simulink model "fangzhen"  (R2022a)
settings: Solver=FixedStepAuto  StartTime=0.0  StopTime=1  FixedStep=0.001  RelTol=1e-3
settings Model: Creator=Userx  LastModifiedBy=Userx

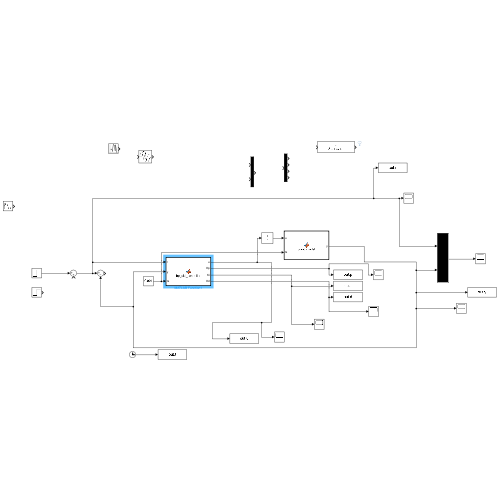
[thumbnail: Simulink's stored preview of the top-level diagram]
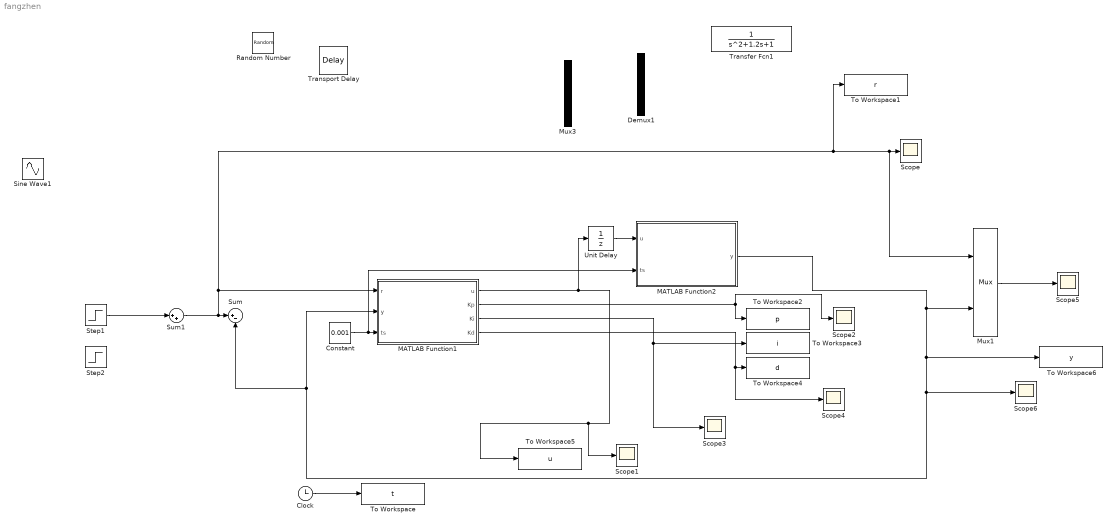
== system fangzhen ==
  Clock : Clock
  Constant : Constant  Value=0.001
  Demux1 : Demux
  MATLAB Function1 : MATLAB Function  TreatAsAtomicUnit=on
  MATLAB Function2 : MATLAB Function  TreatAsAtomicUnit=on
  Mux1 : Mux  Inputs=2
  Mux3 : Mux  Inputs=2
  Random Number : RandomNumber  Variance=0.05  SampleTime=0.1
  Scope{,1..6} (7 alike) : Scope
  Sine Wave1 : Sin  Frequency=5  SampleTime=0
  Step1 : Step  Time=0  SampleTime=0
  Step2 : Step  Time=200  SampleTime=0
  Sum : Sum  Inputs=|+-
  Sum1 : Sum  Inputs=|++
  To Workspace : ToWorkspace  VariableName=t  SampleTime=-1
  To Workspace1 : ToWorkspace  VariableName=r  SampleTime=-1
  To Workspace2 : ToWorkspace  VariableName=p  SampleTime=-1
  To Workspace3 : ToWorkspace  VariableName=i  SampleTime=-1
  To Workspace4 : ToWorkspace  VariableName=d  SampleTime=-1
  To Workspace5 : ToWorkspace  VariableName=u  SampleTime=-1
  To Workspace6 : ToWorkspace  VariableName=y  SampleTime=-1
  Transfer Fcn1 : TransferFcn  Denominator=[1 1.2 1]
  Transport Delay : TransportDelay  DelayTime=0.5
  Unit Delay : UnitDelay  SampleTime=-1  HasFrameUpgradeWarning=on
  wires:
  Mux1/1 -> Scope5/1
  MATLAB Function1/2(Kp) -> Scope2/1, To Workspace2/1
  MATLAB Function1/3(Ki) -> Scope3/1, To Workspace3/1
  MATLAB Function1/4(Kd) -> Scope4/1, To Workspace4/1
  Clock/1 -> To Workspace/1
  Sum1/1 -> MATLAB Function1/1(r), To Workspace1/1, Mux1/1, Scope/1, Sum/1
  MATLAB Function2/1(y) -> MATLAB Function1/2(y), Sum/2, Scope6/1, To Workspace6/1, Mux1/2
  Step1/1 -> Sum1/1
  MATLAB Function1/1(u) -> Unit Delay/1, Scope1/1, To Workspace5/1
  Constant/1 -> MATLAB Function2/2(ts), MATLAB Function1/3(ts)
  Unit Delay/1 -> MATLAB Function2/1(u)

== matlab function fangzhen/MATLAB Function1 ==
  settings: updateMethod=DISCRETE
  data: r input; u output; y input; ts input; Kp output; Ki output; Kd output
function [u, Kp, Ki, Kd] = bp_pid_controller(r, y, ts)
% =========================================================================
%  BP 神经网络 PID 参数自整定控制器
%  用途：放入 Simulink 的 MATLAB Function 模块中使用
%
%  网络结构：
%    输入层  → 3 个神经元：[e(k), Δe(k), Δ²e(k)]
%    隐含层  → 6 个神经元，激活函数：tanh
%    输出层  → 3 个神经元：[Kp, Ki, Kd]，激活函数：sigmoid（保证正值）
%
%  控制律：增量式 PID
%    Δu(k) = Kp·Δe(k) + Ki·ts·e(k) + Kd/ts·Δ²e(k)
%    u(k)  = u(k-1) + Δu(k)
%
%  在线学习：每采样周期执行一次 BP 反向传播 + 带动量项的权值更新
%  Jacobian：采用差商近似 ∂y/∂u ≈ Δy/Δu（符号提取，增强鲁棒性）
%
%  输入：
%    r  - 参考指令（设定值）
%    y  - 被控对象测量输出
%    ts - 采样时间（由外部 Constant 模块接入）
%
%  输出：
%    u  - PID 控制量（输出给被控对象）
%    Kp - 比例系数（用于监控）
%    Ki - 积分系数（用于监控）
%    Kd - 微分系数（用于监控）
%
%  作者：自动生成  版本：v1.0
% =========================================================================

%% ============================= 超参数 ===================================
%  以下常量均可根据被控对象特性自行调整

lr       = 0.0001;   % 学习率：控制每步权值更新幅度，过大震荡，过小收敛慢
alpha    = 0.1;   % 动量系数：加速收敛、抑制震荡，范围建议 [0.01, 0.1]
u_max    = 10.0;    % 控制量上限（防积分饱和 / 执行器限幅）
u_min    = -10.0;   % 控制量下限
Kp_max   = 5.0;    % Kp 的最大允许值（sigmoid 输出乘以此系数）
Ki_max   = 1.0;     % Ki 的最大允许值
Kd_max   = 1.0;     % Kd 的最大允许值

% 神经网络结构参数（修改后需同步修改 persistent 变量维度）
n_in     = 3;       % 输入层神经元数
n_hid    = 6;       % 隐含层神经元数
n_out    = 3;       % 输出层神经元数（固定为 3，对应 Kp/Ki/Kd）

%% ========================== Persistent 变量 =============================
%  所有跨采样周期需要保留的状态均声明为 persistent

% 神经网络权值与偏置
persistent W1 B1    % 隐含层：W1(n_hid × n_in), B1(n_hid × 1)
persistent W2 B2    % 输出层：W2(n_out × n_hid), B2(n_out × 1)

% 动量项（存储上一时刻的权值增量）
persistent dW1_prev dB1_prev
persistent dW2_prev dB2_prev

% 历史误差与控制量（用于计算差分及 Jacobian）
persistent e_k1     % e(k-1)：上一时刻误差
persistent e_k2     % e(k-2)：上上时刻误差
persistent u_k1     % u(k-1)：上一时刻控制量
persistent y_k1     % y(k-1)：上一时刻被控对象输出（Jacobian 估算用）
persistent u_k2 
% 初始化标志
persistent is_init

%% ========================= 首次运行初始化 ================================
 if isempty(is_init)

    % ---- 权值初始化：均匀分布小随机数，打破网络对称性 ----
    W1 = 0.2 * (rand(n_hid, n_in) - 0.5);
    B1 = 0.2 * (rand(n_hid, 1) - 0.5);
    W2 = 0.2 * (rand(n_out, n_hid) - 0.5);
    B2 = 0.2 * (rand(n_out, 1) - 0.5);

%     % ---- 动量增量初始化为零 ----
    dW1_prev = zeros(n_hid, n_in);
    dB1_prev = zeros(n_hid, 1);
    dW2_prev = zeros(n_out, n_hid);
    dB2_prev = zeros(n_out, 1);
% 
%     % ---- 历史状态初始化 ----
    e_k1   = 0;
    e_k2   = 0;
    u_k1   = 0;
    y_k1   = 0;
u_k2 = 0;
    is_init = true;
end



%% ======================= Step 1：误差计算 ================================

e   = r - y;                        % 当前误差 e(k)
de  = e - e_k1;                     % 误差一阶差分 Δe(k) = e(k) - e(k-1)
dde = e - 2.0*e_k1 + e_k2;         % 误差二阶差分 Δ²e(k)（用于 D 项）

%% ======================= Step 2：神经网络前向传播 ========================

% 输入向量（3×1）
x_in = [e; de; dde];

% -- 隐含层计算 --
z1 = W1 * x_in + B1;               % (n_hid × 1)
o1 = tanh(z1);                      % (n_hid × 1)

% -- 输出层计算 --
z2 = W2 * o1 + B2;                 % (n_out × 1)
o2 = 1.0 ./ (1.0 + exp(-z2));      % (n_out × 1)

% 将网络输出映射到实际 PID 参数范围
Kp = Kp_max * o2(1);
Ki = Ki_max * o2(2);
Kd = Kd_max * o2(3);

%% ======================= Step 3：增量式 PID 控制律 ======================

% 增量计算
Ti=0.003;
delta_u = Kp * de  +  Ki * e*0.001 +  Kd * dde;

% 位置累加
u_raw = u_k1 + delta_u;

% -- 积分饱和处理（输出限幅）--
if u_raw > u_max
    u = u_max;
elseif u_raw < u_min
    u = u_min;
else
    u = u_raw;
end

%% ======================= Step 4：Jacobian 估算 ===========================

delta_y_obs  = y   - y_k1;         % Δy = y(k) - y(k-1)
% delta_u_obs  = u   - u_k1;         % Δu = u(k) - u(k-1)
delta_u_obs  = u_k1 - u_k2; 
if abs(delta_u_obs) > 1e-6
    dydu_raw = delta_y_obs / delta_u_obs;
else
    dydu_raw = delta_y_obs * 1e3;
end

jac_sign = sign(dydu_raw);
if jac_sign == 0
    jac_sign = 1;
end

%% ======================= Step 5：BP 反向传播 =============================

dE_du = (-e) * jac_sign;           % ∂E/∂u（标量）

du_do2 = [Kp_max * de;
          Ki_max  *0.001* e;
          Kd_max * (dde)];    % (3×1)

% -- 输出层灵敏度 δ2（3×1）--
sig_grad = o2 .* (1.0 - o2);       % sigmoid 导数
delta2   = dE_du * du_do2 .* sig_grad;

% -- 输出层权值梯度 --
grad_W2 = delta2 * o1';            % (3×6)
grad_B2 = delta2;                  % (3×1)

% -- 隐含层灵敏度 δ1（6×1）--
tanh_grad = 1.0 - o1.^2;          % tanh 导数
delta1    = (W2' * delta2) .* tanh_grad; % (6×1)

% -- 隐含层权值梯度 --
grad_W1 = delta1 * x_in';          % (6×3)
grad_B1 = delta1;                  % (6×1)

%% ======================= Step 6：带动量项的权值更新 =====================

new_dW2 = -lr * grad_W2 + alpha * dW2_prev;
new_dB2 = -lr * grad_B2 + alpha * dB2_prev;
new_dW1 = -lr * grad_W1 + alpha * dW1_prev;
new_dB1 = -lr * grad_B1 + alpha * dB1_prev;

W2 = W2 + new_dW2;
B2 = B2 + new_dB2;
W1 = W1 + new_dW1;
B1 = B1 + new_dB1;

dW2_prev = new_dW2;
dB2_prev = new_dB2;
dW1_prev = new_dW1;
dB1_prev = new_dB1;

%% ======================= Step 7：状态更新 ================================

e_k2 = e_k1;
u_k2 = u_k1;
e_k1 = e;
u_k1 = u;
y_k1 = y;

end

== matlab function fangzhen/MATLAB Function2 ==
  settings: updateMethod=DISCRETE
  data: u input; y output; ts input
function y = plant_model(u, ts)
% =========================================================================
% 非线性时变被控对象
% 模型：y(k) = a(k)/(1+y²(k-1)) * y(k-1) + u(k-1)
%       其中 a(k) = 1.2 * (1 - 0.8*exp(-0.1*k))
% =========================================================================

persistent y_1  k

if isempty(y_1)
    y_1 = 0;
    k   = 0;
end

k = k + 1;

% 时变系数
a_k = 1.2 * (1 - 0.8 * exp(-0.1 * k));

% 计算当前输出
y = a_k / (1 + y_1^2) * y_1 + u;

% 更新状态
y_1 = y;
end
